simulink model "Pitchcontrol_2MW"  (R2020a)
settings: Solver=VariableStepAuto  StartTime=0.0  StopTime=120  RelTol=1e-3  EnableMultiTasking=on
values from neighbouring files (symbols this model uses):
  a1 = 0.5176    [data.mat]
  a2 = 116    [data.mat]
  a3 = 0.4    [data.mat]
  a4 = 5    [data.mat]
  a5 = 21    [data.mat]
  a6 = 0.0068    [data.mat]
  a7 = 0.09    [data.mat]
  a8 = 0.035    [data.mat]
  Ad = 6031.85789489    [data.mat]
  denp = den_P    [Wind_Turbine_Pitch.m]    (also in data.mat = [91260000000000 145900000000000 1.431e+17 7.554e+15 2.279e+1)
  dent = den_P    [Wind_Turbine_Pitch.m]    (also in data.mat = [91260000000000 145900000000000 1.431e+17 7.554e+15 2.279e+1)
  nump = num_P    [Wind_Turbine_Pitch.m]    (also in data.mat = [16590000 26450000 25540000000 6335000000 3680000000000])
  numt = num_T    [Wind_Turbine_Pitch.m]    (also in data.mat = [-75000000 -527900000000 -306700000000000])
  sigma = 1 - Lm^2/(Ls*Lr)    (= 0.0661284179513)    [Generator_specs.m]    (also in data.mat = 0.075)
  Tgd_max = 14000    [Wind_Turbine_Pitch.m]    (also in data.mat)
  Tie = 1    [data.mat]
  Tiu = 10000    [data.mat]
  Tix = 1    [data.mat]
  Tpe = 1    [data.mat]
  Tpu = 10000    [data.mat]
  Tpx = 10000    [data.mat]
undefined symbols (not defined in the file or in its folder): sigbuilder_block
settings Model: Creator=likhi  LastModifiedBy=param
settings DataIOCC: ReturnWorkspaceOutputs=off
settings OptimizationCC: LifeSpan=inf
settings DebuggingCC: SFUnexpectedBacktrackingDiag=warning  SFNoUnconditionalDefaultTransitionDiag=warning  SFExecutionAtInitializationDiag=none  ArithmeticOperatorsInVariantConditions=warning
settings SFSimCC: SimUseLocalCustomCode=off  CustomCodeUndefinedFunction=UseInterfaceOnly
settings RTWCC: RTWUseLocalCustomCode=off
settings CodeAppCC: StateflowObjectComments=on
settings GRTTargetCC: TargetLangStandard=C89/C90 (ANSI)
settings ConfigComp: CovMetricSettings=dw  CovHtmlReporting=on  CovSaveCumulativeToWorkspaceVar=on  CovSaveSingleToWorkspaceVar=on  CovExternalEMLEnable=off

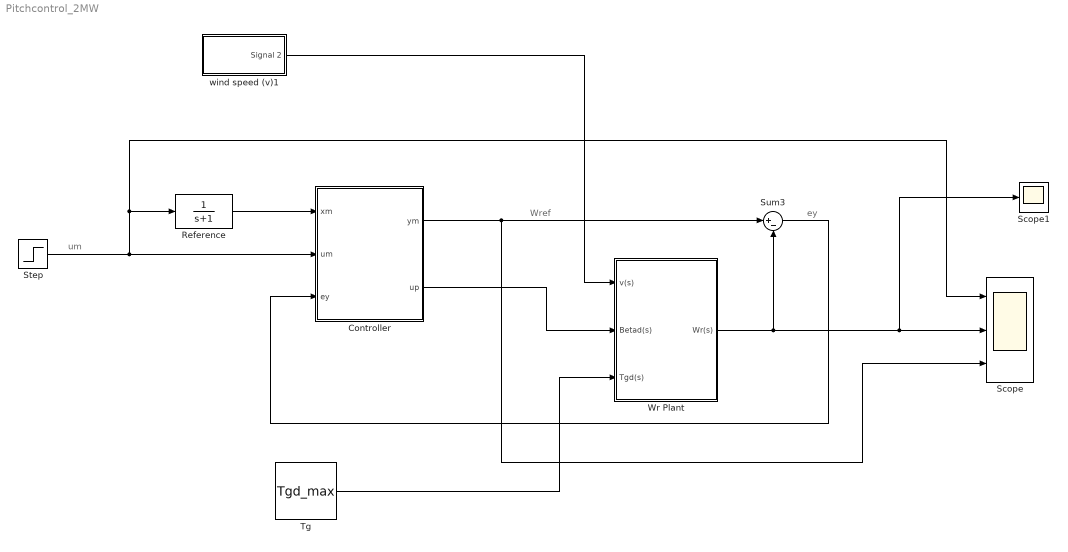
== system Pitchcontrol_2MW ==
  note: um
  note: ey
  note: Wref
  Controller : Subsystem
  Reference : TransferFcn  Denominator=[1 1]
  Scope : Scope  NumInputPorts=3
  Scope1 : Scope
  Step : Step  Time=0  After=2  SampleTime=0
  Sum3 : Sum  Inputs=|+-
  Tg : Constant  Value=Tgd_max
  Wr Plant : Subsystem
  wind speed (v)1 : Subsystem  Tag=STV Subsys  LoadFcn=sigbuilder_block('load');  StartFcn=sigbuilder_block('start');  StopFcn=sigbuilder_block('stop');  ClipboardFcn=sigbuilder_block('clipboard');  mask(Sigbuilder block){tuvar=[0:10]}
      mask help: Simulink:masks:SigbuilderBlock_MD
      mask init:
      | if ~strcmp(get_param(bdroot(gcbh),'SimulationStatus'),'stopped') tuvar = sigbuilder_block('maskInit'); end
      settings: CopyFcn=sigbuilder_block('copy');  DeleteFcn=sigbuilder_block('delete');  ModelCloseFcn=sigbuilder_block('modelClose');  PreSaveFcn=sigbuilder_block('preSave');  PauseFcn=sigbuilder_block('pause');  ContinueFcn=sigbuilder_block('continue');  NameChangeFcn=sigbuilder_block('namechange');  OpenFcn=sigbuilder_block('open',[289.8 114 442.2 307.8 ]);  CloseFcn=sigbuilder_block('close');
      mask Display: plot(0, 0, 100, 100,[2, 2, 32, 32, 2], [68, 8, 8, 68, 68],[32, 2], [38, 38], [32, 19, 2],[53, 60, 44], [32, 17, 17, 2],[16, 16, 31, 31]);txt = getActiveGroup(gcbh);text(2, 100, txt,'verticalAlignment', 'top');
  wires:
  Controller/2(up) -> Wr Plant/2(Betad(s))
  Wr Plant/1(Wr(s)) -> Scope1/1, Scope/2, Sum3/2
  Tg/1 -> Wr Plant/3(Tgd(s))
  wind speed (v)1/1(Signal 2) -> Wr Plant/1(v(s))
  Sum3/1 -> Controller/3(ey)
  Reference/1 -> Controller/1(xm)
  Step/1 -> Scope/1, Reference/1, Controller/2(um)
  Controller/1(ym) -> Scope/3, Sum3/1

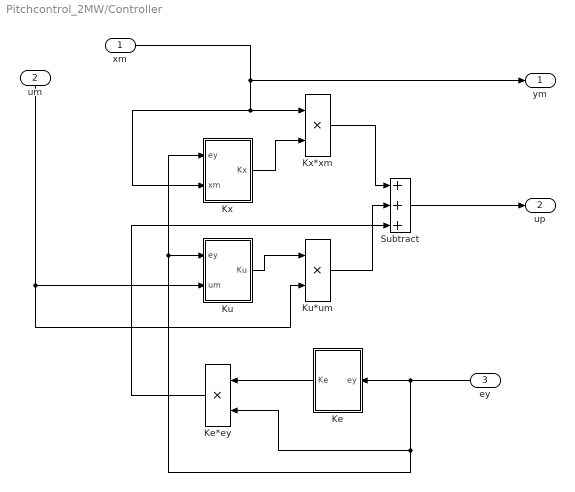
== system Pitchcontrol_2MW/Controller ==
  xm : Inport
  um : Inport  Port=2
  ey : Inport  Port=3
  Ke : Subsystem
  Ke*ey : Product
  Ku : Subsystem
  Ku*um : Product
  Kx : Subsystem
  Kx*xm : Product
  Subtract : Sum  Inputs=+++
  ym : Outport
  up : Outport  Port=2
  wires:
  Kx/1(Kx) -> Kx*xm/2
  Ke/1(Ke) -> Ke*ey/1
  Ku*um/1 -> Subtract/2
  Kx*xm/1 -> Subtract/1
  xm/1 -> Kx*xm/1, Kx/2(xm), ym/1
  ey/1 -> Kx/1(ey), Ku/1(ey), Ke*ey/2, Ke/1(ey)
  Ku/1(Ku) -> Ku*um/1
  Ke*ey/1 -> Subtract/3
  um/1 -> Ku/2(um), Ku*um/2
  Subtract/1 -> up/1

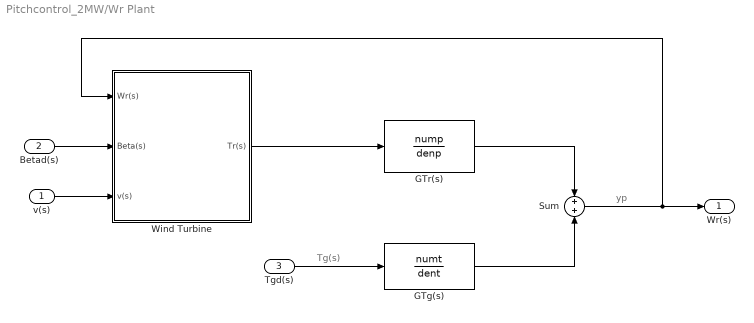
== system Pitchcontrol_2MW/Wr Plant ==
  note: yp
  note: Tg(s)
  v(s) : Inport
  Betad(s) : Inport  Port=2
  Tgd(s) : Inport  Port=3
  GTg(s) : TransferFcn  Numerator=numt  Denominator=dent
  GTr(s) : TransferFcn  Numerator=nump  Denominator=denp
  Sum : Sum
  Wind Turbine : Subsystem  AncestorBlock=re_lib/Wind Generation/Wind Turbine  DialogController=POWERSYS.PowerSysDialog  mask(Wind Turbine){Pnom=2e6, Pelec_base=2e6/0.9, wind_base=9, P_wind_base=0.73, speed_nom=1.2, pitch_angle=10, c1_c6=[0.51763          116          0.4            5           21     0.006795], cp_nom=0.48, lambda_nom=8.1}
      mask prompts: Pnom "Nominal mechanical output power (W):"; Pelec_base "Base power of the electrical generator (VA):"; wind_base "Base wind speed (m/s):"; P_wind_base "Maximum power at base wind speed (pu of nominal mechanical power):"; speed_nom "Base rotational speed (p.u. of base generator speed):"; pitch_angle "Pitch angle beta to display wind-turbine power characteristics (beta >=0)  (deg):"
      mask help:
      | This block implements a variable pitch wind turbine model. The performance coefficient Cp of the turbine is the mechanical output power of the turbine divided by wind power and a function of wind speed, rotational speed, and pitch angle (beta). Cp reaches its maximum value at zero beta. Select the wind-turbine power characteristics display to plot the turbine characteristics at the specified pitch angle.
      |
      | The first input is the generator speed in per unit of the generator base speed. For a synchronous or asynchronous generator, the base speed is the synchronous speed. For a permanent-magnet generator, the base speed is defined as the speed producing nominal voltage at  no load. The second input is the blade pitch angle (beta) in degrees. The third input is the wind speed in m/s.
      |
      | The output is the torque applied to the generator shaft in per unit of the generator ratings.
      |
      | The turbine inertia must be added to the generator inertia.
      mask init:
      | c1=c1_c6(1);c2=c1_c6(2);c3=c1_c6(3);c4=c1_c6(4);c5=c1_c6(5);c6=c1_c6(6);
      | power_initmask();
      mask Help: helpview(psbhelp);
      mask DialogControl DisplayTurbChar Prompt: Display wind turbine power characteristics
      mask DialogControl DisplayTurbChar Callback: WindTurbinePlot(gcb)
      mask Display: disp('');
  Wr(s) : Outport
  wires:
  v(s)/1 -> Wind Turbine/3(v(s))
  Sum/1 -> Wind Turbine/1(Wr(s)), Wr(s)/1
  Tgd(s)/1 -> GTg(s)/1
  GTg(s)/1 -> Sum/2
  GTr(s)/1 -> Sum/1
  Betad(s)/1 -> Wind Turbine/2(Beta(s))
  Wind Turbine/1(Tr(s)) -> GTr(s)/1

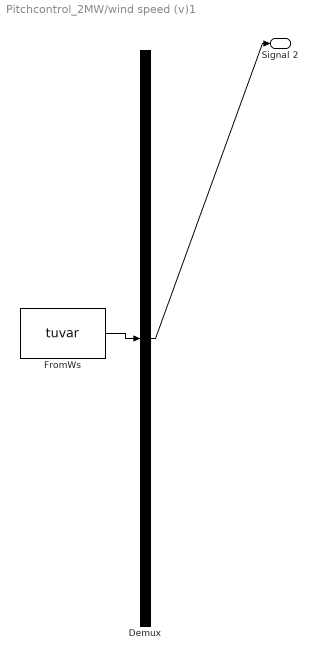
== system Pitchcontrol_2MW/wind speed (v)1 ==
  Demux : Demux  Tag=STV Demux  Outputs=1
      settings: DisplayOption=none
  FromWs : FromWorkspace  Tag=STV FromWs  VariableName=tuvar
      SigBuilderData=|
      | common.afterFinalStr = 'Extrapolate'
      | common.sampleTime = 0
      | dataSet(1).timeRange = [0 120]
      | dataSet(1).name = 'Group 1'
      | dataSet(2).timeRange = [0 120]
      | dataSet(2).name = 'Group 2'
      | sbobj.Groups(1).Name = 'Group 1'
      | sbobj.Groups(1).Signals.Name = 'Signal 2'
      | sbobj.Groups(1).Signals.XData = [0 0.1 0.2 0.3 0.4 0.5 0.6 0.7 0.8 0.9 1 1.1 ... (1201 elements, 1x1201)]
      | sbobj.Groups(1).Signals.YData = [15.5376671395 16.8338850146 12.741153139 15.8621733204 15.3187652399 13.6923117037 14.5664079777 15.3426244665 18.5783969397 17.7694370299 13.6501130598 18.0349234663 ... (1201 elements, 1x1201)]
      | sbobj.Groups(1).TimeRange = [0 120]
      | sbobj.Groups(2).Name = 'Group 2'
      | sbobj.Groups(2).Signals.Name = 'Signal 2'
      | sbobj.Groups(2).Signals.XData = [0 0.5 1 1.5 2 2.5 3 3.5 4 4.5 5 5.5 6 6.5 7 7.5 8 8.5 9 9.5 10 10.5 11 11.5 12 12.5 13 13.5 14 14.5 15 15.5 16 16.5 17 17.5 18 18.5 19 19.5 20 20.5 21 21.5 22 22.5 23 23.5 24 24.5 25 25.5 26 26.5 27 27.5 28 28.5 29 29.5 30 30.5 31 31.5 32 32.5 33 33.5 34 34.5 35 35.5 36 36.5 37 37.5 38 38.5 39 39.5 40 40.5 41 41.5 42 42.5 43 43.5 44 44.5 45 45.5 46 46.5 47 47.5 48 48.5 49 49.5 50 50.5 51 51.5 52 52.5 53 53.5 54 54.5 55 55.5 56 56.5 57 57.5 58 58.5 59 59.5 60 60.5 61 61.5 62 62.5 63 63.5 64 64.5 65 65.5 66 66.5 67 67.5 68 68.5 69 69.5 70 70.5 71 71.5 72 72.5 73 73.5 74 74.5 75 75.5 76 76.5 77 77.5 78 78.5 79 79.5 80 80.5 81 81.5 82 82.5 83 83.5 84 84.5 85 85.5 86 86.5 87 87.5 88 88.5 89 89.5 90 90.5 91 91.5 92 92.5 93 93.5 94 94.5 95 95.5 96 96.5 97 97.5 98 98.5 99 99.5 100 100.5 101 101.5 102 102.5 103 103.5 104 104.5 105 105.5 106 106.5 107 107.5 108 108.5 109 109.5 110 110.5 111 111.5 112 112.5 113 113.5 114 114.5 115 115.5 116 116.5 117 117.5 118 118.5 119 119.5 120]
      | sbobj.Groups(2).Signals.YData = [14.0719772886 16.4017514434 16.5838938847 15.2403409151 15.4311004804 15.9493583656 12.8114371964 14.1274354118 12.2547760168 14.3263453802 16.4239120554 16.0761621142 ... (241 elements, 1x241)]
      | sbobj.Groups(2).TimeRange = [0 120]
  Signal 2 : Outport  Tag=STV Outport
  wires:
  Demux/1 -> Signal 2/1
  FromWs/1 -> Demux/1

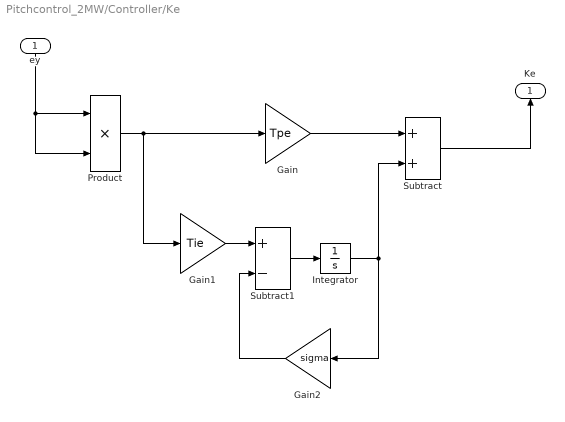
== system Pitchcontrol_2MW/Controller/Ke ==
  ey : Inport
  Gain : Gain  Gain=Tpe
  Gain1 : Gain  Gain=Tie
  Gain2 : Gain  Gain=sigma
  Integrator : Integrator
  Product : Product
  Subtract : Sum
  Subtract1 : Sum  Inputs=+-
  Ke : Outport
  wires:
  Subtract/1 -> Ke/1
  ey/1 -> Product/2, Product/1
  Product/1 -> Gain1/1, Gain/1
  Gain/1 -> Subtract/1
  Gain1/1 -> Subtract1/1
  Subtract1/1 -> Integrator/1
  Integrator/1 -> Gain2/1, Subtract/2
  Gain2/1 -> Subtract1/2

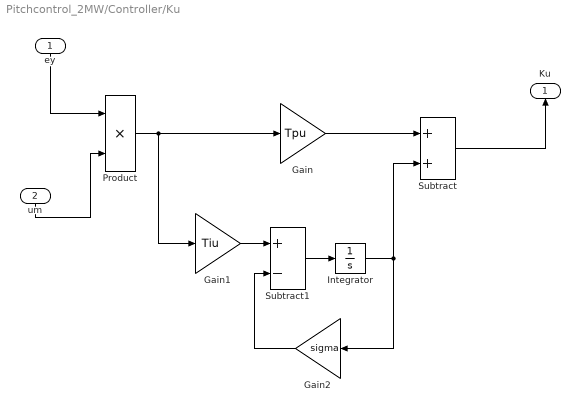
== system Pitchcontrol_2MW/Controller/Ku ==
  ey : Inport
  um : Inport  Port=2
  Gain : Gain  Gain=Tpu
  Gain1 : Gain  Gain=Tiu
  Gain2 : Gain  Gain=sigma
  Integrator : Integrator
  Product : Product
  Subtract : Sum
  Subtract1 : Sum  Inputs=+-
  Ku : Outport
  wires:
  Gain2/1 -> Subtract1/2
  Integrator/1 -> Subtract/2, Gain2/1
  Subtract1/1 -> Integrator/1
  Gain1/1 -> Subtract1/1
  Gain/1 -> Subtract/1
  Product/1 -> Gain/1, Gain1/1
  Subtract/1 -> Ku/1
  ey/1 -> Product/1
  um/1 -> Product/2

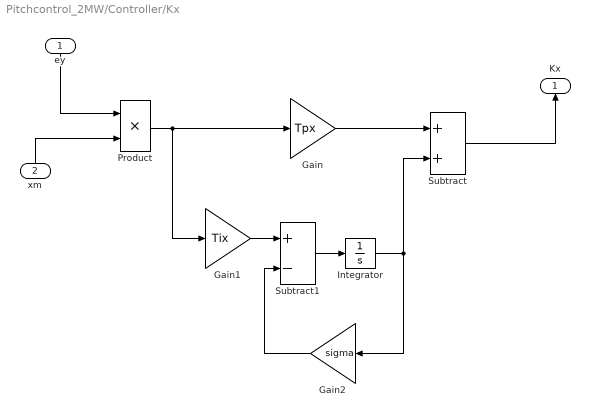
== system Pitchcontrol_2MW/Controller/Kx ==
  ey : Inport
  xm : Inport  Port=2
  Gain : Gain  Gain=Tpx
  Gain1 : Gain  Gain=Tix
  Gain2 : Gain  Gain=sigma
  Integrator : Integrator
  Product : Product
  Subtract : Sum
  Subtract1 : Sum  Inputs=+-
  Kx : Outport
  wires:
  Subtract/1 -> Kx/1
  Gain/1 -> Subtract/1
  Gain1/1 -> Subtract1/1
  Subtract1/1 -> Integrator/1
  Integrator/1 -> Gain2/1, Subtract/2
  Gain2/1 -> Subtract1/2
  Product/1 -> Gain1/1, Gain/1
  ey/1 -> Product/1
  xm/1 -> Product/2

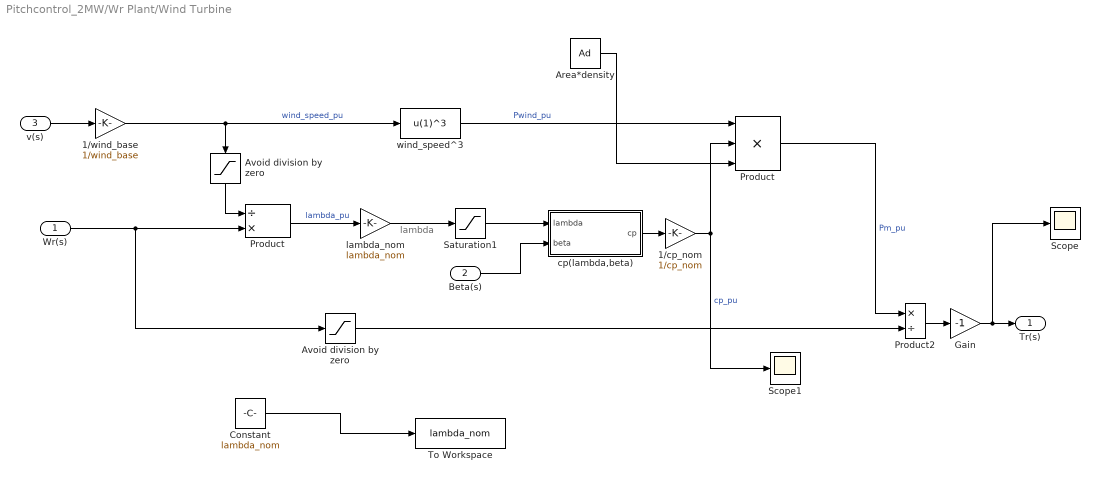
== system Pitchcontrol_2MW/Wr Plant/Wind Turbine ==
  note: lambda
  Wr(s) : Inport
  Beta(s) : Inport  Port=2
  v(s) : Inport  Port=3
  1/cp_nom : Gain  Gain=1/cp_nom  SaturateOnIntegerOverflow=on  OutDataTypeStr=Inherit: Same as input  ParamDataTypeStr=Inherit: Same as input
  1/wind_base : Gain  Gain=1/wind_base  SaturateOnIntegerOverflow=on  OutDataTypeStr=Inherit: Same as input  ParamDataTypeStr=Inherit: Same as input
  Area*density : Constant  Value=Ad
  Avoid division by zero : Saturate  UpperLimit=1e6  LowerLimit=1e-6
  "Avoid division by zero " : Saturate  UpperLimit=1e6  LowerLimit=1e-6
  Constant : Constant  Value=lambda_nom
  Gain : Gain  Gain=-1  SaturateOnIntegerOverflow=on  OutDataTypeStr=Inherit: Same as input  ParamDataTypeStr=Inherit: Same as input
  Product : Product  Inputs=/*  SaturateOnIntegerOverflow=on  OutDataTypeStr=Inherit: Same as first input
  "Product " : Product  Inputs=3  SaturateOnIntegerOverflow=on  OutDataTypeStr=Inherit: Same as first input
  Product2 : Product  Inputs=*/  InputSameDT=on  SaturateOnIntegerOverflow=on  OutDataTypeStr=Inherit: Same as first input
  Saturation1 : Saturate  UpperLimit=inf  LowerLimit=1e-6
  Scope : Scope
  Scope1 : Scope
  To Workspace : ToWorkspace  VariableName=lambda_nom  SaveFormat=Timeseries  SampleTime=-1
  cp(lambda,beta) : Subsystem
  lambda_nom : Gain  Gain=lambda_nom  SaturateOnIntegerOverflow=on  OutDataTypeStr=Inherit: Same as input  ParamDataTypeStr=Inherit: Same as input
  wind_speed^3 : Fcn  Expr=u(1)^3
  Tr(s) : Outport
  wires:
  Area*density/1 -> "Product "/3
  Wr(s)/1 -> Avoid division by zero/1, Product/2
  "Avoid division by zero "/1 -> Product/1
  1/wind_base/1 -> "Avoid division by zero "/1, wind_speed^3/1  "wind_speed_pu"
  Product/1 -> lambda_nom/1  "lambda_pu"
  Saturation1/1 -> cp(lambda,beta)/1(lambda)
  1/cp_nom/1 -> "Product "/2, Scope1/1  "cp_pu"
  lambda_nom/1 -> Saturation1/1
  "Product "/1 -> Product2/1  "Pm_pu"
  v(s)/1 -> 1/wind_base/1
  Avoid division by zero/1 -> Product2/2
  Product2/1 -> Gain/1
  wind_speed^3/1 -> "Product "/1  "Pwind_pu"
  cp(lambda,beta)/1(cp) -> 1/cp_nom/1
  Beta(s)/1 -> cp(lambda,beta)/2(beta)
  Gain/1 -> Scope/1, Tr(s)/1
  Constant/1 -> To Workspace/1

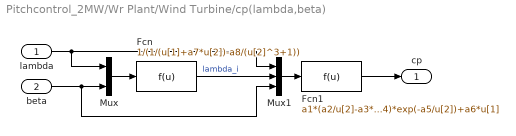
== system Pitchcontrol_2MW/Wr Plant/Wind Turbine/cp(lambda,beta) ==
  lambda : Inport
  beta : Inport  Port=2
  Fcn : Fcn  Expr=1/(1/(u[1]+a7*u[2])-a8/(u[2]^3+1))
  Fcn1 : Fcn  Expr=a1*(a2/u[2]-a3*u[3]-a4)*exp(-a5/u[2])+a6*u[1]
  Mux : Mux  Inputs=2
  Mux1 : Mux  Inputs=3
  cp : Outport
  wires:
  Mux/1 -> Fcn/1
  beta/1 -> Mux/2, Mux1/3
  Mux1/1 -> Fcn1/1
  lambda/1 -> Mux/1, Mux1/1
  Fcn1/1 -> cp/1
  Fcn/1 -> Mux1/2  "lambda_i"
